simulink model "Simple_Joystick_Controller"  (R2025b)
settings: Solver=VariableStepAuto  StartTime=0.0  StopTime=10.0  RelTol=1e-3
libraries: ros2lib x3
settings Model: Creator=vulcangrip  LastModifiedBy=vulcangrip

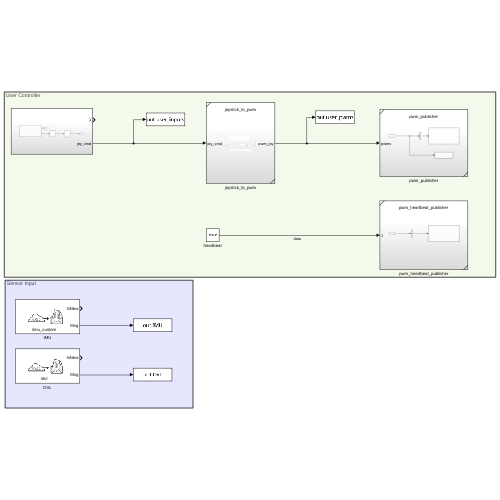
[thumbnail: Simulink's stored preview of the top-level diagram]
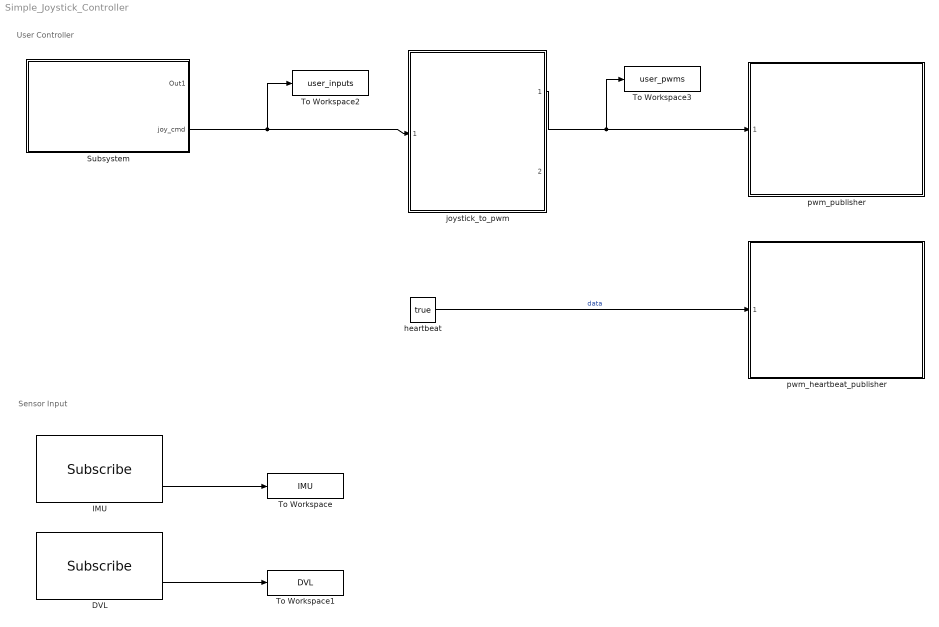
== system Simple_Joystick_Controller ==
  note: User Controller
  note: Sensor Input
  DVL : ros2lib/Subscribe  topicSource=Specify your own  topic=/dvl  messageType=custom_interfaces/Position  sampleTime=-1  QOSHistory=Keep last  QOSDepth=10  QOSReliability=Reliable  QOSDurability=Volatile  QOSDeadline=Inf  QOSLifespan=Inf  QOSLiveliness=Automatic  QOSLeaseDuration=Inf  QOSAvoidROSNamespaceConventions=off
  IMU : ros2lib/Subscribe  topicSource=Specify your own  topic=/imu_custom  messageType=custom_interfaces/Imu  sampleTime=-1  QOSHistory=Keep last  QOSDepth=10  QOSReliability=Reliable  QOSDurability=Volatile  QOSDeadline=Inf  QOSLifespan=Inf  QOSLiveliness=Automatic  QOSLeaseDuration=Inf  QOSAvoidROSNamespaceConventions=off
  Subsystem : Subsystem
  To Workspace : ToWorkspace  VariableName=IMU  SaveFormat=Timeseries  SampleTime=-1
  To Workspace1 : ToWorkspace  VariableName=DVL  SaveFormat=Timeseries  SampleTime=-1
  To Workspace2 : ToWorkspace  VariableName=user_inputs  SaveFormat=Timeseries  SampleTime=-1
  To Workspace3 : ToWorkspace  VariableName=user_pwms  SaveFormat=Timeseries  SampleTime=-1
  heartbeat : Constant  Value=true
  joystick_to_pwm : Subsystem  ReferencedSubsystem=joystick_to_pwm
  pwm_heartbeat_publisher : Subsystem  ReferencedSubsystem=pwm_heartbeat_publisher
  pwm_publisher : Subsystem  ReferencedSubsystem=pwm_publisher
  wires:
  Subsystem/2(joy_cmd) -> To Workspace2/1, joystick_to_pwm/1
  joystick_to_pwm/1 -> To Workspace3/1, pwm_publisher/1
  heartbeat/1 -> pwm_heartbeat_publisher/1  "data"
  IMU/2 -> To Workspace/1
  DVL/2 -> To Workspace1/1

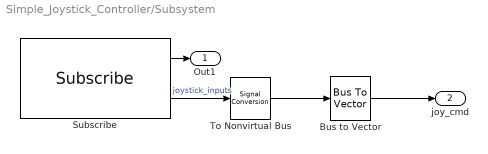
== system Simple_Joystick_Controller/Subsystem ==
  Bus to Vector : BusToVector
  Subscribe : ros2lib/Subscribe  topicSource=Specify your own  topic=/ps5_controller  messageType=remote_control_interface/Gamepad  sampleTime=1/60  QOSHistory=Keep last  QOSDepth=10  QOSReliability=Reliable  QOSDurability=Volatile  QOSDeadline=Inf  QOSLifespan=Inf  QOSLiveliness=Automatic  QOSLeaseDuration=Inf  QOSAvoidROSNamespaceConventions=off
  To Nonvirtual Bus : SignalConversion  ConversionOutput=Virtual bus  OverrideOpt=off
  Out1 : Outport
  joy_cmd : Outport  Port=2
  wires:
  To Nonvirtual Bus/1 -> Bus to Vector/1
  Subscribe/2 -> To Nonvirtual Bus/1  "joystick_inputs"
  Subscribe/1 -> Out1/1
  Bus to Vector/1 -> joy_cmd/1
